simulink model "workflow"  (R2015a)
settings: Solver=ode45  StartTime=0.0  StopTime=10  RelTol=1e-3
settings Model: Creator=Frank  LastModifiedBy=Frank

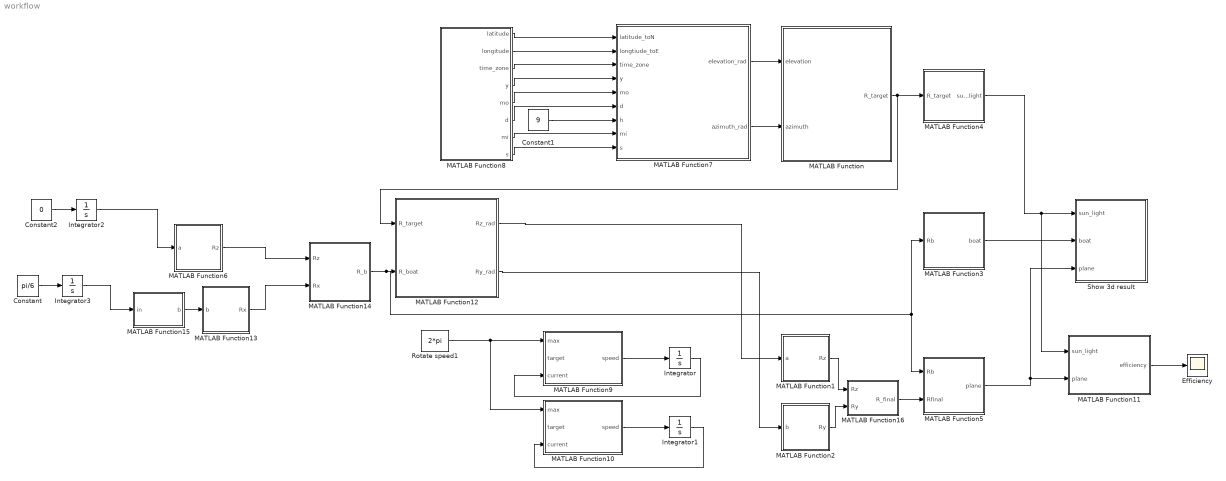
== system workflow ==
  Constant : Constant  Value=pi/6
  Constant1 : Constant  Value=9
  Constant2 : Constant  Value=0
  Efficiency : Scope
      settings: TimeRange=11  YMin=0  YMax=1  SaveName=ScopeData2
  Integrator{,1..3} (4 alike) : Integrator
  MATLAB Function : MATLAB Function  TreatAsAtomicUnit=on
  MATLAB Function1 : MATLAB Function  TreatAsAtomicUnit=on
  MATLAB Function10 : MATLAB Function  TreatAsAtomicUnit=on
  MATLAB Function11 : MATLAB Function  TreatAsAtomicUnit=on
  MATLAB Function12 : MATLAB Function  TreatAsAtomicUnit=on
  MATLAB Function13 : MATLAB Function  TreatAsAtomicUnit=on
  MATLAB Function14 : MATLAB Function  TreatAsAtomicUnit=on
  MATLAB Function15 : MATLAB Function  TreatAsAtomicUnit=on
  MATLAB Function16 : MATLAB Function  TreatAsAtomicUnit=on
  MATLAB Function2 : MATLAB Function  TreatAsAtomicUnit=on
  MATLAB Function3 : MATLAB Function  TreatAsAtomicUnit=on
  MATLAB Function4 : MATLAB Function  TreatAsAtomicUnit=on
  MATLAB Function5 : MATLAB Function  TreatAsAtomicUnit=on
  MATLAB Function6 : MATLAB Function  TreatAsAtomicUnit=on
  MATLAB Function7 : MATLAB Function  TreatAsAtomicUnit=on
  MATLAB Function8 : MATLAB Function  TreatAsAtomicUnit=on
  MATLAB Function9 : MATLAB Function  TreatAsAtomicUnit=on
  Rotate speed1 : Constant  Value=2*pi
  Show 3d result : MATLAB Function  TreatAsAtomicUnit=on
  wires:
  MATLAB Function/1(R_target) -> MATLAB Function4/1(R_target), MATLAB Function12/1(R_target)
  MATLAB Function4/1(sun_light) -> MATLAB Function11/1(sun_light), Show 3d result/1(sun_light)
  MATLAB Function5/1(plane) -> Show 3d result/3(plane), MATLAB Function11/2(plane)
  MATLAB Function3/1(boat) -> Show 3d result/2(boat)
  MATLAB Function8/1(latitude) -> MATLAB Function7/1(latitude_toN)
  MATLAB Function8/2(longitude) -> MATLAB Function7/2(longtiude_toE)
  MATLAB Function8/3(time_zone) -> MATLAB Function7/3(time_zone)
  MATLAB Function8/4(y) -> MATLAB Function7/4(y)
  MATLAB Function8/5(mo) -> MATLAB Function7/5(mo)
  MATLAB Function8/6(d) -> MATLAB Function7/6(d)
  MATLAB Function8/7(mi) -> MATLAB Function7/8(mi)
  MATLAB Function8/8(s) -> MATLAB Function7/9(s)
  MATLAB Function7/2(azimuth_rad) -> MATLAB Function/2(azimuth)
  Rotate speed1/1 -> MATLAB Function9/1(max), MATLAB Function10/1(max)
  MATLAB Function9/1(speed) -> Integrator/1
  Integrator/1 -> MATLAB Function9/3(current)
  MATLAB Function10/1(speed) -> Integrator1/1
  Integrator1/1 -> MATLAB Function10/3(current)
  MATLAB Function14/1(R_b) -> MATLAB Function5/1(Rb), MATLAB Function3/1(Rb), MATLAB Function12/2(R_boat)
  MATLAB Function7/1(elevation_rad) -> MATLAB Function/1(elevation)
  MATLAB Function11/1(efficiency) -> Efficiency/1
  MATLAB Function6/1(Rz) -> MATLAB Function14/1(Rz)
  MATLAB Function13/1(Rx) -> MATLAB Function14/2(Rx)
  MATLAB Function15/1(b) -> MATLAB Function13/1(b)
  Constant1/1 -> MATLAB Function7/7(h)
  MATLAB Function1/1(Rz) -> MATLAB Function16/1(Rz)
  MATLAB Function2/1(Ry) -> MATLAB Function16/2(Ry)
  MATLAB Function12/1(Rz_rad) -> MATLAB Function1/1(a)
  MATLAB Function12/2(Ry_rad) -> MATLAB Function2/1(b)
  Constant2/1 -> Integrator2/1
  Integrator2/1 -> MATLAB Function6/1(a)
  Constant/1 -> Integrator3/1
  Integrator3/1 -> MATLAB Function15/1(in)
  MATLAB Function16/1(R_final) -> MATLAB Function5/2(Rfinal)

== matlab function workflow/MATLAB Function2 ==
  data: b input; Ry output
function Ry = rotate_y(b)
Ry = [cos(b) 0 sin(b);0 1 0;-sin(b) 0 cos(b)];
end

== matlab function workflow/MATLAB Function1 ==
  data: a input; Rz output
function Rz = rotate_z(a)
Rz = [cos(a) -sin(a) 0;sin(a) cos(a) 0;0 0 1];
end

== matlab function workflow/MATLAB Function4 ==
  data: R_target input; sun_light output
function sun_light = get_sun_light(R_target)
%#codegen
vector = [0 0;0 0;1 8];
sun_light = R_target*vector;
end

== matlab function workflow/MATLAB Function ==
  data: elevation input; R_target output; azimuth input
function R_target = get_target(elevation,azimuth)

a = 2*pi - azimuth;
b = pi/2 - elevation;
Rz = [cos(a) -sin(a) 0;sin(a) cos(a) 0;0 0 1];
Ry = [cos(b) 0 sin(b);0 1 0;-sin(b) 0 cos(b)];
R_target = Rz*Ry;
end

== matlab function workflow/MATLAB Function3 ==
  data: Rb input; boat output
function boat = get_boat(Rb)
w=5;
boat = [-w -w 1.5*w;-w w 0;0 0 0];
boat = Rb*boat;
boat = boat - [0 0 0;0 0 0;8 8 8];
end

== matlab function workflow/MATLAB Function5 ==
  data: Rb input; plane output; Rfinal input
function plane = get_plane(Rb,Rfinal)
%#codegen
R0 = Rb*Rfinal;
w = 5;
plane = [w w -w -w;w -w -w w;0 0 0 0];
plane = R0*plane;
end

== matlab function workflow/Show 3d result ==
  data: sun_light input; boat input; plane input
function draw(sun_light,boat,plane)
%#codegen

x_p = plane(1,:);
y_p = plane(2,:);
z_p = plane(3,:);
fill3(x_p,y_p,z_p,z_p/10+0.5);
hold on
x_b = boat(1,:);
y_b = boat(2,:);
z_b = boat(3,:);
fill3(x_b,y_b,z_b,'g');
hold off
hold on
x_s = sun_light(1,:);
y_s = sun_light(2,:);
z_s = sun_light(3,:);
fill3(x_s,y_s,z_s,'b');
hold off
xlim([-12 12]);
ylim([-12 12]);
zlim([-12 12]);
xlabel('X, North');
ylabel('Y, West');
zlabel('Z');
daspect([1 1 1]);

end

== matlab function workflow/MATLAB Function6 ==
  data: a input; Rz output
function Rz = rotate_z(a)
Rz = [cos(a) -sin(a) 0;sin(a) cos(a) 0;0 0 1];
end

== matlab function workflow/MATLAB Function7 ==
  data: latitude_toN input; longtiude_toE input; time_zone input; y input; elevation_rad output; azimuth_rad output; mo input; d input; h input; mi input; s input
function [elevation_rad, azimuth_rad] = Solar_Angle_Calculation...
    (latitude_toN,longtiude_toE,time_zone,y,mo,d,h,mi,s)
%   This function caculate the elevation angle
%   Detailed explanation goes here
julian_day = julian_date(y,mo,d,h,mi,s);
julian_century = (julian_day-2451545)/36525;
geom_mean_long_sun = mod(280.46646+julian_century*...
    (36000.76983+julian_century*0.0003032),360);
geom_mean_anom_sun = 357.52911+julian_century*...
    (35999.05029-0.0001537*julian_century);
eccent_earth_orbit = 0.016708634-julian_century*...
    (0.000042037+0.0000001267*julian_century);
sun_eq_of_ctr = sin(deg2rad(geom_mean_anom_sun))*...
    (1.914602-julian_century*(0.004817+0.000014*julian_century))+...
    sin(deg2rad(2*geom_mean_anom_sun))*...
    (0.019993-0.000101*julian_century)+...
    sin(deg2rad(3*geom_mean_anom_sun))*0.000289;
sun_true_long = geom_mean_long_sun + sun_eq_of_ctr;
sun_true_anom = geom_mean_anom_sun + sun_eq_of_ctr;
%disp(sun_true_long);
%disp(sun_true_anom);
mean_obliq_ecliptic = 23+(26+((21.448-julian_century*...
    (46.815+julian_century*(0.00059-julian_century*0.001813))))/60)/60;
obliq_corr = mean_obliq_ecliptic+0.00256*...
    cos(deg2rad(125.04-1934.136*julian_century));
sun_app_long = sun_true_long-0.00569-0.00478*...
    sin(deg2rad(125.04-1934.136*julian_century));
var_y = tan(deg2rad(obliq_corr/2))*tan(deg2rad(obliq_corr/2));
sun_declin = rad2deg(asin(sin(deg2rad(obliq_corr))*...
    sin(deg2rad(sun_app_long))));
eq_of_time = 4*rad2deg(var_y*sin(2*deg2rad(geom_mean_long_sun))...
    -2*eccent_earth_orbit*sin(deg2rad(geom_mean_anom_sun))...
    +4*eccent_earth_orbit*var_y*sin(deg2rad(geom_mean_anom_sun))...
    *cos(2*deg2rad(geom_mean_long_sun))...
    -0.5*var_y*var_y*sin(4*deg2rad(geom_mean_long_sun))...
    -1.25*eccent_earth_orbit*eccent_earth_orbit*sin(2*deg2rad(geom_mean_anom_sun)));
%disp(eq_of_time);
time_past_midnight = h/24 + mi/1440 + s/86400;
true_solar_time = mod(time_past_midnight*1440+eq_of_time+4*longtiude_toE-60*time_zone,1440);
if true_solar_time/4 <0
    hour_angle = true_solar_time/4+180;
else
    hour_angle = true_solar_time/4-180;
end
solar_zenith_angle = rad2deg(acos(sin(deg2rad(latitude_toN))*sin(deg2rad(sun_declin))+...
    cos(deg2rad(latitude_toN))*cos(deg2rad(sun_declin))*cos(deg2rad(hour_angle))));
elevation_deg = 90 - solar_zenith_angle;
if hour_angle > 0
    azimuth_deg = mod(rad2deg(acos(((sin(deg2rad(latitude_toN))*cos(deg2rad(solar_zenith_angle)))-...
        sin(deg2rad(sun_declin)))/(cos(deg2rad(latitude_toN))*sin(deg2rad(solar_zenith_angle)))))+180,360);
else
    azimuth_deg = mod(540-rad2deg(acos(((sin(deg2rad(latitude_toN))*cos(deg2rad(solar_zenith_angle)))-...
        sin(deg2rad(sun_declin)))/(cos(deg2rad(latitude_toN))*sin(deg2rad(solar_zenith_angle))))),360);
end
elevation_rad = deg2rad(elevation_deg);
azimuth_rad = deg2rad(azimuth_deg);
%disp(elevation_rad);
%disp(azimuth_rad);
end
function rad=deg2rad(deg)
rad = double(deg)/180*pi;
end
function deg=rad2deg(rad)
deg = double(rad)/pi*180;
end
function julian_day = julian_date(y,mo,d,h,mi,s)
julian_day_number = (1461*(y + 4800 + (mo - 14)/12))/4 +(367*(mo - 2 - 12 * ((mo - 14)/12)))/12 -...
    (3 * ((y + 4900 + (mo - 14)/12)/100))/4 + d - 32075;
julian_day = julian_day_number + (h-12)/24 + mi/1440 + s/86400;
end

== matlab function workflow/MATLAB Function8 ==
  data: latitude output; longitude output; time_zone output; y output; mo output; d output; mi output; s output
function [latitude,longitude,time_zone,y,mo,d,mi,s] = data_feeder()
% coder.extrinsic('format');
% coder.extrinsic('clock');
latitude = 22;
longitude = 114;
time_zone = 8;
y=2017;
mo=4;
d=16;
h=7;
mi=0;
s=0;
% format shortg
% c = clock;
% fix(c);
% y = c(0);
% mo = c(1);
% d = c(2);
% h = c(3);
% mi = c(4);
% s = c(5);

end

== matlab function workflow/MATLAB Function9 ==
  data: max input; target input; speed output; current input
function speed = set_speed(max,target,current)
%#codegen
target = mod(target,2*pi);
current = mod(current,2*pi);
if abs(target-current) >0.01
    if and (current >= 0, current < pi)
        if and(target > current,target <= current + pi)
            speed = abs(max);
        else
            speed = -abs(max);
        end
    else
        if or(target>current, target<= mod(current+pi,2*pi))
            speed = abs(max);
        else
            speed = -abs(max);
        end
    end
else
    speed = 0;
end
end

== matlab function workflow/MATLAB Function10 ==
  data: max input; target input; speed output; current input
function speed = set_speed(max,target,current)
%#codegen
target = mod(target,2*pi);
current = mod(current,2*pi);
if abs(target-current) >0.01
    if and (current >= 0, current < pi)
        if and(target > current,target <= current + pi)
            speed = abs(max);
        else
            speed = -abs(max);
        end
    else
        if or(target>current, target<= mod(current+pi,2*pi))
            speed = abs(max);
        else
            speed = -abs(max);
        end
    end
else
    speed = 0;
end
end

== matlab function workflow/MATLAB Function11 ==
  data: sun_light input; efficiency output; plane input
function efficiency = efficient_analysis(sun_light,plane)
%#codegen
v1 = plane(:,1)-plane(:,2);
v2 = plane(:,2)-plane(:,3);
z = 1;
temp = v1(2)*v2(1)-v2(2)*v1(1);
x = (-v1(2)*v2(3)+v2(2)*v1(3))/temp;
efficiency = (-v1(3)*v2(1)+v2(3)*v1(1))/temp;
n = [x efficiency z];
sun_direction = sun_light(:,2) - sun_light(:,1);
efficiency = n*sun_direction/(norm(n)*norm(sun_direction));

== matlab function workflow/MATLAB Function12 ==
  data: R_target input; R_boat input; Rz_rad output; Ry_rad output
function [Rz_rad,Ry_rad] = set_angle(R_target,R_boat)
%#codegen
R_modify = R_boat\R_target;
Rz_rad = atan2(R_modify(2,3),R_modify(1,3));
Ry_rad = atan2(R_modify(2,3),R_modify(3,3)*sin(Rz_rad));
% Rz_boat = atan2(R_boat(2,1),R_boat(1,1));
% Rx_boat = atan2(R_boat(3,2),R_boat(3,3));
% Ry_rad = atan2(-R_target(3,1),R_target(3,3));
% Rz_rad = atan2(-R_target(1,2),R_target(2,2));

Ry_rad = mod(Ry_rad,2*pi);
if Ry_rad > pi
    Ry_rad = 2*pi - Ry_rad;
    Rz_rad = Rz_rad + pi;
end
Rz_rad = mod(Rz_rad,2*pi);
end

== matlab function workflow/MATLAB Function13 ==
  data: b input; Rx output
function Rx = rotate_x(b)
Rx = [1 0 0; 0 cos(b) -sin(b); 0 sin(b) cos(b)];
end

== matlab function workflow/MATLAB Function14 ==
  data: Rz input; R_b output; Rx input
function R_b = boat_rotate(Rz,Rx)
%#codegen

R_b = Rz*Rx;

== matlab function workflow/MATLAB Function15 ==
  data: in input; b output
function b = Rx_controller(in)
%#codegen
rotate_limit = pi/4;
temp = mod(in,4*rotate_limit);
b = temp;
if and (temp >=0, temp<rotate_limit)
    b = temp;
end
if and (temp >=rotate_limit, temp<3*rotate_limit)
    b = 2*rotate_limit - temp;
end
if temp >=3*rotate_limit
    b = temp - 4*rotate_limit;
end

end

== matlab function workflow/MATLAB Function16 ==
  data: Rz input; R_final output; Ry input
function R_final = multiply(Rz,Ry)
%#codegen
R_final = Rz * Ry;
end
